simulink model "ACC_System"  (R2024b)
settings: Solver=VariableStepAuto  StartTime=0.0  StopTime=inf  RelTol=1e-3
(part 2 of 2)

== stateflow chart ACC_System/ACC_Logic ==
  state FOLLOWING
    %busy road
    entry:
    State_Display = 2;
    during:
    Accel_Req = 0;
    % On freine si on est trop près
    Brake_Req = true;
  state OFF
    entry:
    Accel_Req = 0;
    Brake_Req = false;
    State_Display = 0;
  state CRUISING
    %Clear road
    entry:
    State_Display = 1;
    during:
    Brake_Req = false;
    %  on accélère si on est trop lent
    Accel_Req = (Set_Speed - Current_Speed) * 2;
  (default) -> OFF
  FOLLOWING -> OFF [order 2] : [Switch_ACC == 0]
  FOLLOWING -> CRUISING [order 1] : [Radar_Dist > 60]
  CRUISING -> FOLLOWING [order 2] : [Radar_Dist < 50]
  OFF -> CRUISING : [Switch_ACC == 1]
  CRUISING -> OFF [order 1] : [Switch_ACC == 0]
  data: Switch_ACC input boolean; Current_Speed input uint8; Radar_Dist input uint8; Accel_Req output uint8; Brake_Req output boolean; State_Display output uint8; Set_Speed input
